simulink model "EE2_RetourEtat"  (R2012b)
settings: Solver=ode45  StartTime=0.0  StopTime=2  RelTol=1e-4
values from neighbouring files (symbols this model uses):
  K = [0 K(2)]    [CommandeEE2.m]
undefined symbols (not defined in the file or in its folder): EE0, EE1, EE2, EE2_bf, obsver
settings Model: Creator=Lucien  LastModifiedBy=David
settings OptimizationCC: ExpressionDepthLimit=128
settings DebuggingCC: UnderspecifiedInitializationDetection=Simplified  MergeDetectMultiDrivingBlocksExec=error  SolverPrmCheckMsg=none  FrameProcessingCompatibilityMsg=error  StateNameClashWarn=none
settings CodeAppCC: CustomSymbolStrType=$N$R$M_T
settings GRTTargetCC: CodeReplacementLibrary=C89/C90 (ANSI)

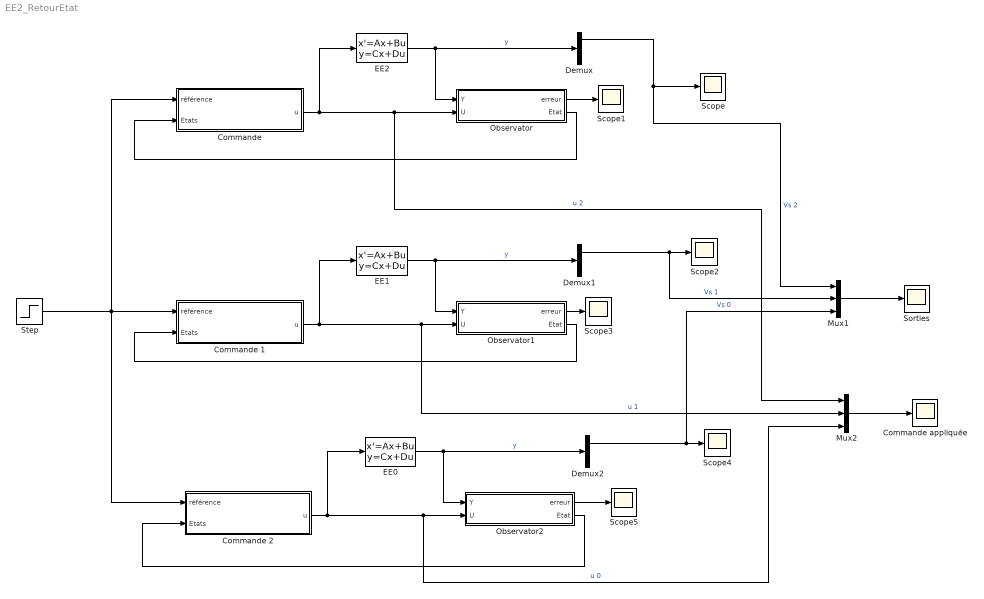
== system EE2_RetourEtat ==
  "Commande " : Subsystem
  Commande 1 : Subsystem
  Commande 2 : Subsystem
  Commande appliquée : Scope
      settings: YMin=3.31  YMax=3.54  SaveName=ScopeData10
  Demux : Demux  Outputs=2
  Demux1 : Demux  Outputs=2
  Demux2 : Demux  Outputs=2
  EE0 : StateSpace  A=EE0.ee.a  B=EE0.ee.b  C=EE0.ee.c  D=EE0.ee.d  X0=0
  EE1 : StateSpace  A=EE1.ee.a  B=EE1.ee.b  C=EE1.ee.c  D=EE1.ee.d  X0=0
  "EE2 " : StateSpace  A=EE2.ee.a  B=EE2.ee.b  C=EE2.ee.c  D=EE2.ee.d  X0=0
  Mux1 : Mux  Inputs=3
  Mux2 : Mux  Inputs=3
  Observator : Subsystem
  Observator1 : Subsystem
  Observator2 : Subsystem
  Scope{,1..5} (6 alike) : Scope
      Scope settings: YMin=0.33855  YMax=0.3391  SaveName=ScopeData3
      Scope1 settings: SaveName=ScopeData4
      Scope2 settings: YMin=0.33855  YMax=0.3391  SaveName=ScopeData5
      Scope3 settings: SaveName=ScopeData6
      Scope4 settings: YMin=0.33855  YMax=0.3391  SaveName=ScopeData7
      Scope5 settings: SaveName=ScopeData8
  Sorties : Scope
      settings: YMin=0.33855  YMax=0.3391  SaveName=ScopeData9
  "Step " : Step  Time=0  After=5  SampleTime=0
  wires:
  "EE2 "/1 -> Observator/1("Y "), Demux/1  "y"
  Observator/1(erreur) -> Scope1/1
  Demux/1 -> Scope/1, Mux1/1  "Vs 2"
  Observator/2("Etat ") -> "Commande "/2(Etats)
  EE1/1 -> Observator1/1("Y "), Demux1/1  "y"
  Observator1/1(erreur) -> Scope3/1
  Demux1/1 -> Mux1/2, Scope2/1  "Vs 1"
  Observator1/2("Etat ") -> Commande 1/2(Etats)
  "Step "/1 -> "Commande "/1(référence), Commande 1/1(référence), Commande 2/1(référence)
  EE0/1 -> Observator2/1("Y "), Demux2/1  "y"
  Observator2/1(erreur) -> Scope5/1
  Demux2/1 -> Scope4/1, Mux1/3  "Vs 0"
  Observator2/2("Etat ") -> Commande 2/2(Etats)
  Mux1/1 -> Sorties/1
  "Commande "/1(u) -> Mux2/1, Observator/2(U), "EE2 "/1  "u 2"
  Commande 1/1(u) -> Mux2/2, Observator1/2(U), EE1/1  "u 1"
  Commande 2/1(u) -> Mux2/3, Observator2/2(U), EE0/1  "u 0"
  Mux2/1 -> Commande appliquée/1

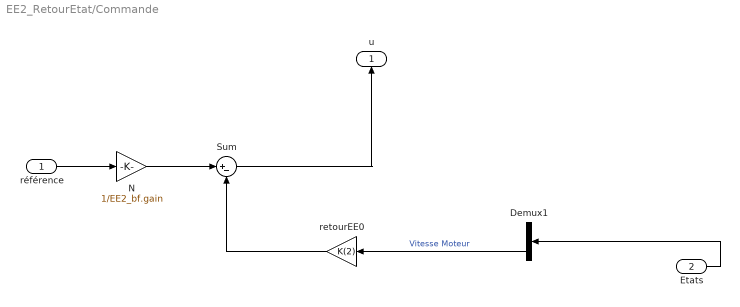
== system EE2_RetourEtat/Commande  ==
  référence : Inport
  Etats : Inport  Port=2
  Demux1 : Demux  Outputs=2
  "N " : Gain  Gain=1/EE2_bf.gain
  Sum : Sum  Inputs=|+-
  retourEE0 : Gain  Gain=K(2)
  u : Outport
  wires:
  Sum/1 -> u/1
  référence/1 -> "N "/1
  Etats/1 -> Demux1/1
  retourEE0/1 -> Sum/2
  "N "/1 -> Sum/1
  Demux1/2 -> retourEE0/1  "Vitesse Moteur"

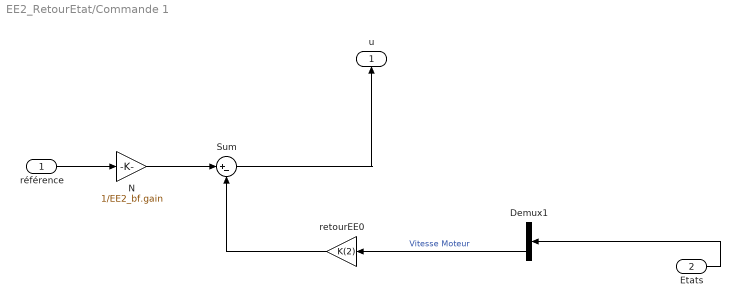
== system EE2_RetourEtat/Commande 1 ==
  référence : Inport
  Etats : Inport  Port=2
  Demux1 : Demux  Outputs=2
  "N " : Gain  Gain=1/EE2_bf.gain
  Sum : Sum  Inputs=|+-
  retourEE0 : Gain  Gain=K(2)
  u : Outport
  wires:
  Sum/1 -> u/1
  référence/1 -> "N "/1
  Etats/1 -> Demux1/1
  retourEE0/1 -> Sum/2
  "N "/1 -> Sum/1
  Demux1/2 -> retourEE0/1  "Vitesse Moteur"

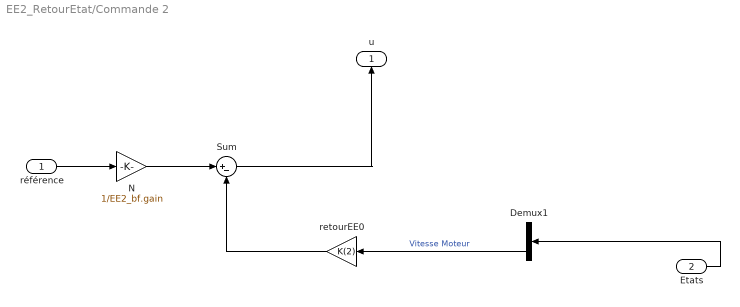
== system EE2_RetourEtat/Commande 2 ==
  référence : Inport
  Etats : Inport  Port=2
  Demux1 : Demux  Outputs=2
  "N " : Gain  Gain=1/EE2_bf.gain
  Sum : Sum  Inputs=|+-
  retourEE0 : Gain  Gain=K(2)
  u : Outport
  wires:
  Sum/1 -> u/1
  référence/1 -> "N "/1
  Etats/1 -> Demux1/1
  retourEE0/1 -> Sum/2
  "N "/1 -> Sum/1
  Demux1/2 -> retourEE0/1  "Vitesse Moteur"

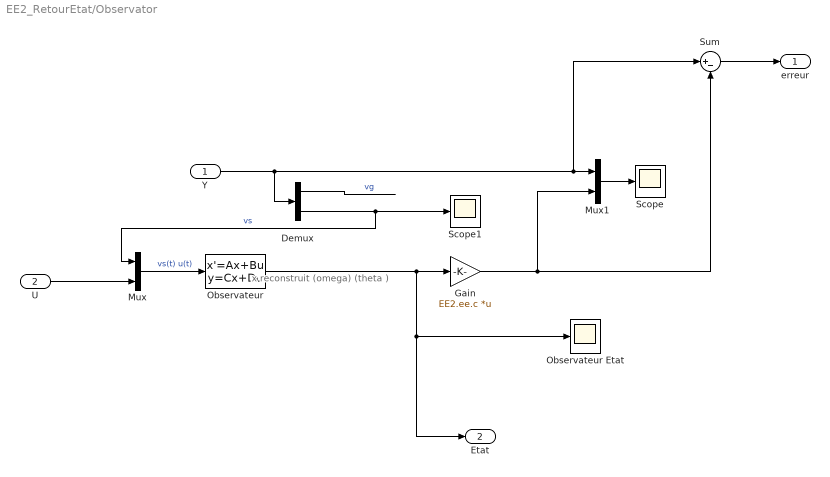
== system EE2_RetourEtat/Observator ==
  note: x reconstruit
      | (omega)
      | (theta   )
  "Y " : Inport
  U : Inport  Port=2
  Demux : Demux  Outputs=2
  Gain : Gain  Gain=EE2.ee.c  Multiplication=Matrix(K*u)
  Mux : Mux  Inputs=2
  Mux1 : Mux  Inputs=2
  "Observateur " : StateSpace  A=obsver.ee.a  B=obsver.ee.b  C=obsver.ee.c  D=obsver.ee.d  X0=0
  "Observateur Etat " : Scope
  Scope : Scope
      settings: YMin=-1  YMax=1
  Scope1 : Scope
      settings: YMin=16  YMax=30  SaveName=ScopeData2
  Sum : Sum  Inputs=|+-
  erreur : Outport
  "Etat " : Outport  Port=2
  wires:
  Mux1/1 -> Scope/1
  "Observateur "/1 -> "Etat "/1, "Observateur Etat "/1, Gain/1
  Demux/2 -> Mux/1, Scope1/1  "vs"
  Sum/1 -> erreur/1
  Demux/1 -> ?  "vg"
  "Y "/1 -> Sum/1, Mux1/1, Demux/1
  Mux/1 -> "Observateur "/1  "vs(t) u(t)"
  Gain/1 -> Mux1/2, Sum/2
  U/1 -> Mux/2

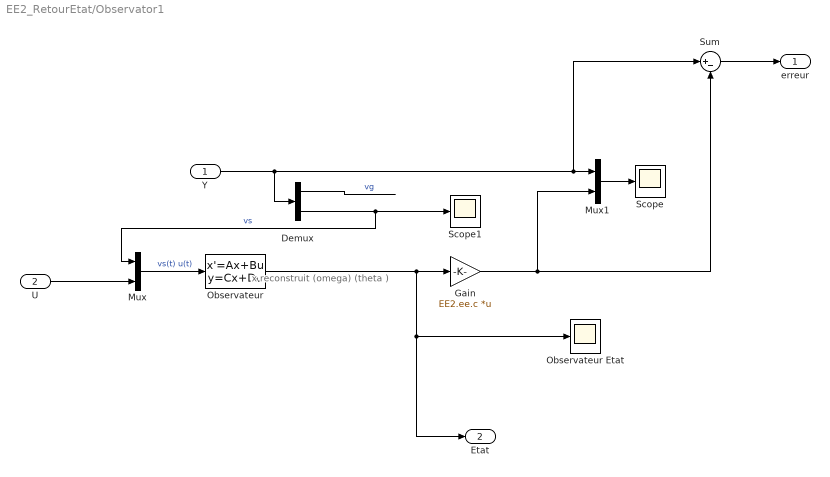
== system EE2_RetourEtat/Observator1 ==
  note: x reconstruit
      | (omega)
      | (theta   )
  "Y " : Inport
  U : Inport  Port=2
  Demux : Demux  Outputs=2
  Gain : Gain  Gain=EE2.ee.c  Multiplication=Matrix(K*u)
  Mux : Mux  Inputs=2
  Mux1 : Mux  Inputs=2
  "Observateur " : StateSpace  A=obsver.ee.a  B=obsver.ee.b  C=obsver.ee.c  D=obsver.ee.d  X0=0
  "Observateur Etat " : Scope
  Scope : Scope
      settings: YMin=-1  YMax=1
  Scope1 : Scope
      settings: YMin=16  YMax=30  SaveName=ScopeData2
  Sum : Sum  Inputs=|+-
  erreur : Outport
  "Etat " : Outport  Port=2
  wires:
  Mux1/1 -> Scope/1
  "Observateur "/1 -> "Etat "/1, "Observateur Etat "/1, Gain/1
  Demux/2 -> Mux/1, Scope1/1  "vs"
  Sum/1 -> erreur/1
  Demux/1 -> ?  "vg"
  "Y "/1 -> Sum/1, Mux1/1, Demux/1
  Mux/1 -> "Observateur "/1  "vs(t) u(t)"
  Gain/1 -> Mux1/2, Sum/2
  U/1 -> Mux/2

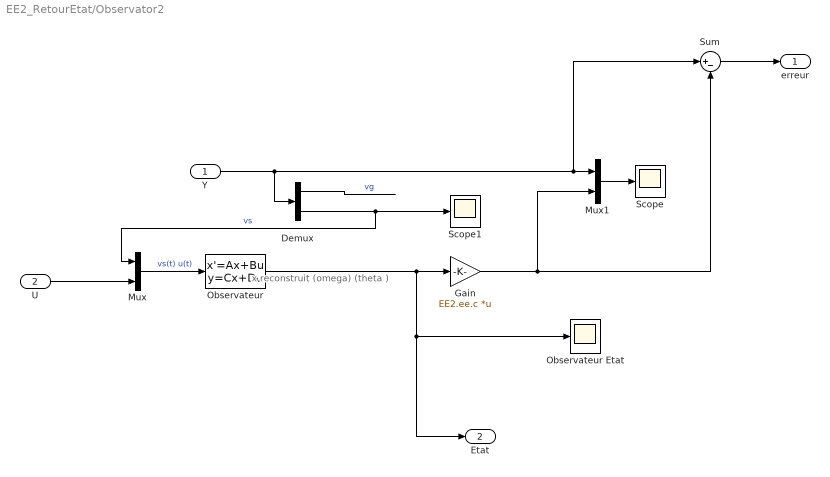
== system EE2_RetourEtat/Observator2 ==
  note: x reconstruit
      | (omega)
      | (theta   )
  "Y " : Inport
  U : Inport  Port=2
  Demux : Demux  Outputs=2
  Gain : Gain  Gain=EE2.ee.c  Multiplication=Matrix(K*u)
  Mux : Mux  Inputs=2
  Mux1 : Mux  Inputs=2
  "Observateur " : StateSpace  A=obsver.ee.a  B=obsver.ee.b  C=obsver.ee.c  D=obsver.ee.d  X0=0
  "Observateur Etat " : Scope
  Scope : Scope
      settings: YMin=-1  YMax=1
  Scope1 : Scope
      settings: YMin=16  YMax=30  SaveName=ScopeData2
  Sum : Sum  Inputs=|+-
  erreur : Outport
  "Etat " : Outport  Port=2
  wires:
  Mux1/1 -> Scope/1
  "Observateur "/1 -> "Etat "/1, "Observateur Etat "/1, Gain/1
  Demux/2 -> Mux/1, Scope1/1  "vs"
  Sum/1 -> erreur/1
  Demux/1 -> ?  "vg"
  "Y "/1 -> Sum/1, Mux1/1, Demux/1
  Mux/1 -> "Observateur "/1  "vs(t) u(t)"
  Gain/1 -> Mux1/2, Sum/2
  U/1 -> Mux/2
